simulink model "adc_demo"  (Simulink 9.2)
settings: Solver=VariableStepDiscrete  StartTime=0.0  StopTime=1  RelTol=1e-3  EnableMultiTasking=on
libraries: simulink_extras x1
settings Model: Creator=rcheng  LastModifiedBy=Acer
settings OptimizationCC: ExpressionDepthLimit=2147483647  InitFltsAndDblsToZero=on
settings DebuggingCC: SolverPrmCheckMsg=warning  LibraryContextMissingDiagnostic=none
settings ConfigComp: CovSFcnEnable=off

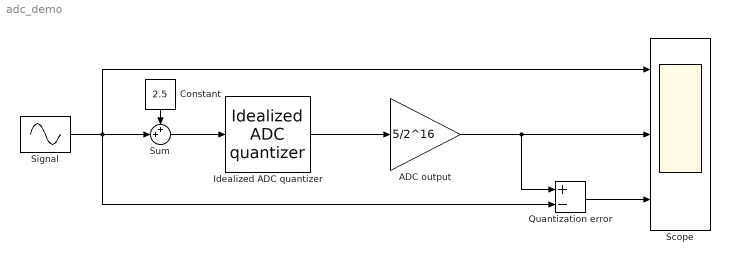
== system adc_demo ==
  ADC output : Gain  Gain=5/2^16
  Constant : Constant  Value=2.5
  Idealized ADC quantizer : simulink_extras/Additional Discrete/Idealized ADC quantizer  NumberOfConverterBits=16  Vmin=0  Vmax=5  OutputDataType=int16  OutputNegativeValues=on
      settings: SourceProductName=Simulink
  Quantization error : Sum  Inputs=+-
  Scope : Scope  NumInputPorts=3
  Signal : Sin  Amplitude=2.5  Frequency=2*pi*100  SampleTime=1/10000
  Sum : Sum  Inputs=++|
  wires:
  Quantization error/1 -> Scope/3
  Idealized ADC quantizer/1 -> ADC output/1
  ADC output/1 -> Quantization error/1, Scope/2
  Signal/1 -> Sum/2, Quantization error/2, Scope/1
  Sum/1 -> Idealized ADC quantizer/1
  Constant/1 -> Sum/1
